simulink model "car_model_with_controller_2020a"  (R2020b)
settings: Solver=ode45  StartTime=0.0  StopTime=170  RelTol=1e-3
values from neighbouring files (symbols this model uses):
  d = 1.1    [constants.m]    (also in navigation.m = 0.64)
  Energy_budget = 1000*input("Define the energy budget(Kj): ")    [constants.m]
  J = 0.0025    [constants.m]
  Kb = 0.06    [constants.m]
  kd = 0    [constants.m]
  ki = 100    [constants.m]
  kp = 70    [constants.m]
  Kt = 11.43    [constants.m]
  l = 0.64    [constants.m]
  L = 0.125    [constants.m]    (also in navigation.m = 2.2)
  m = 810    [constants.m]
  N = 1000    [constants.m]
  P0 = 20    [constants.m]
  r = 0.256    [constants.m]    (also in navigation.m)
  R = 0.688    [constants.m]    (also in kin_controller.m = @(theta) [cos(theta),sin(theta),0;-sin(theta),cos(theta),0;0)
  T = trajectory.tSamples(2)    [constants.m]
  theta_init = atan2(ydot,xdot)    [constants.m]
  x_final = trajectory.q(1,end)    [constants.m]
  x_init = trajectory.q(1,1)    [constants.m]
  y_final = trajectory.q(2,end)    [constants.m]
  y_init = trajectory.q(2,1)    [constants.m]
libraries: simulink x2, pid_lib x2
settings Model: Creator=Tiago  LastModifiedBy=francisco
settings DebuggingCC: SFMachineParentedDataDiag=error  UnderSpecifiedDimensionMsg=warning

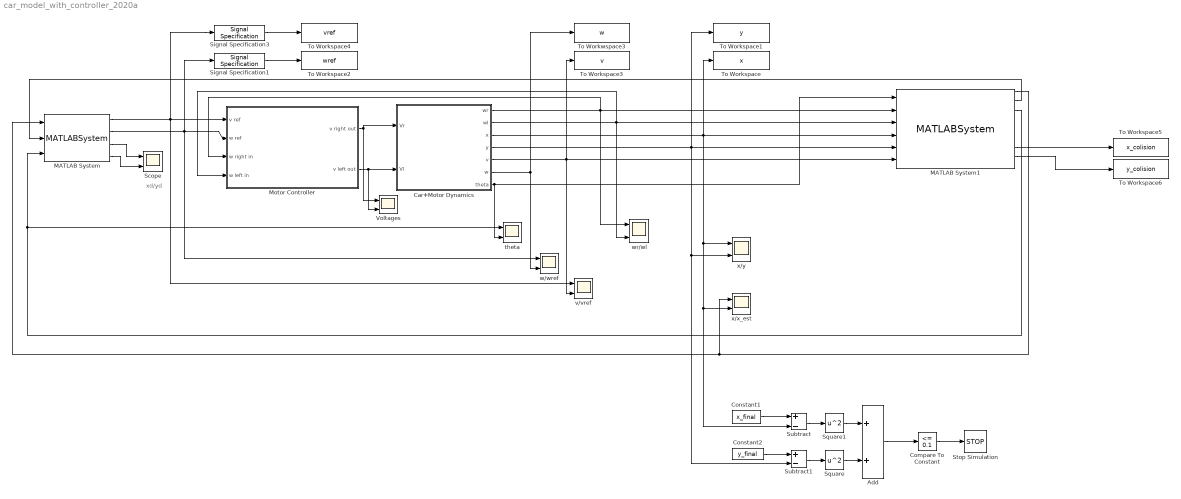
== system car_model_with_controller_2020a ==
  note: xd/yd
  Add : Sum
  Car+Motor Dynamics : Subsystem
  Compare To Constant : simulink/Logic and Bit Operations/Compare To Constant  relop=<=  const=0.1  OutDataTypeStr=boolean
  Constant1 : Constant  Value=x_final
  Constant2 : Constant  Value=y_final
  MATLAB System : MATLABSystem  System=kin_controller  traj=trajectory  OffsetTime=0.0  SampleTime=T  useKinematicModel=false  useFeedback=true  SimulateUsing=Code generation
      mask Type: kin_controller
      mask Display:
      | disp('kin_controller');
      | port_label('input',1,'x');
      | port_label('input',2,'y');
      | port_label('input',3,'theta');
      | port_label('output',1,'v');
      | port_label('output',2,'omega');
      | port_label('output',3,'xd');
      | port_label('output',4,'yd');
  MATLAB System1 : MATLABSystem  System=navigation  initial_x=x_init  initial_y=y_init  initial_theta=theta_init  q_gain=0.001  r_gain=5  OffsetTime=0.0  SampleTime=0.01  position_noise=2  orientation_noise=0.001  angular_speed_noise=0.001  oc_matx=oc_matx  d=0.64  L=2.2  Lr=0.566  Lf=0.566  k=0.1852  SimulateUsing=Code generation
      mask Type: navigation
      mask Display:
      | disp('navigation');
      | port_label('input',1,'theta_measured');
      | port_label('input',2,'omega_r');
      | port_label('input',3,'omega_l');
      | port_label('input',4,'x_real');
      | port_label('input',5,'y_real');
      | port_label('input',6,'V');
      | port_label('output',1,'x');
      | port_label('output',2,'y');
      | port_label('output',3,'theta');
      | port_label('output',4,'x_measured');
      | port_label('output',5,'y_measured');
      | port_label('output',6,'c_check');
      | port_label('output',7,'x_col');
      | port_label('output',8,'y_col');
      | port_label('output',9,'GPS');
  Motor Controller : Subsystem
  Scope : Scope  NumInputPorts=2
  Signal Specification1 : SignalSpecification  Dimensions=1
  Signal Specification3 : SignalSpecification  Dimensions=1
  Square : Math  Operator=square  SaturateOnIntegerOverflow=on
  Square1 : Math  Operator=square  SaturateOnIntegerOverflow=on
  Stop Simulation : Stop
  Subtract : Sum  Inputs=+-
  Subtract1 : Sum  Inputs=+-
  To Workspace : ToWorkspace  VariableName=x  SaveFormat=Timeseries  SampleTime=-1
  To Workspace1 : ToWorkspace  VariableName=y  SaveFormat=Timeseries  SampleTime=-1
  To Workspace2 : ToWorkspace  VariableName=wref  SaveFormat=Timeseries  SampleTime=-1
  To Workspace3 : ToWorkspace  VariableName=v  SaveFormat=Timeseries  SampleTime=-1
  To Workspace4 : ToWorkspace  VariableName=vref  SaveFormat=Timeseries  SampleTime=-1
  To Workspace5 : ToWorkspace  VariableName=x_colision  SampleTime=-1
      settings: Save2DSignal=2-D array (concatenate along first dimension)
  To Workspace6 : ToWorkspace  VariableName=y_colision  SampleTime=-1
      settings: Save2DSignal=2-D array (concatenate along first dimension)
  To Workwspace3 : ToWorkspace  VariableName=w  SaveFormat=Timeseries  SampleTime=-1
  Voltages : Scope  NumInputPorts=2
  theta : Scope  NumInputPorts=2
  v/vref : Scope  NumInputPorts=2
  w/wref : Scope  NumInputPorts=2
  wr/wl : Scope  NumInputPorts=2
  x/x_est : Scope  NumInputPorts=2
  x/y : Scope  NumInputPorts=2
  wires:
  Motor Controller/2(v left out) -> Car+Motor Dynamics/2(Vl), Voltages/2
  Motor Controller/1(v right out) -> Car+Motor Dynamics/1(Vr), Voltages/1
  MATLAB System1/3 -> MATLAB System/3, theta/1
  MATLAB System1/1 -> x/x_est/1, MATLAB System/1
  MATLAB System1/2 -> MATLAB System/2
  Car+Motor Dynamics/1(wr) -> wr/wl/1, MATLAB System1/2, Motor Controller/3(w right in)
  Car+Motor Dynamics/2(wl) -> wr/wl/2, MATLAB System1/3, Motor Controller/4(w left in)
  Car+Motor Dynamics/3(x) -> x/y/1, Subtract/2, x/x_est/2, MATLAB System1/4, To Workspace/1
  Car+Motor Dynamics/4(y) -> x/y/2, Subtract1/2, MATLAB System1/5, To Workspace1/1
  Car+Motor Dynamics/5(v) -> v/vref/2, MATLAB System1/6, To Workspace3/1
  Car+Motor Dynamics/6(w) -> w/wref/2, To Workwspace3/1
  Car+Motor Dynamics/7(theta) -> MATLAB System1/1, theta/2
  MATLAB System/1 -> v/vref/1, Motor Controller/1(v ref), Signal Specification3/1
  MATLAB System/2 -> w/wref/1, Signal Specification1/1, Motor Controller/2(w ref)
  MATLAB System/3 -> Scope/1
  MATLAB System/4 -> Scope/2
  Constant1/1 -> Subtract/1
  Constant2/1 -> Subtract1/1
  Subtract1/1 -> Square/1
  Subtract/1 -> Square1/1
  Compare To Constant/1 -> Stop Simulation/1
  Square1/1 -> Add/1
  Square/1 -> Add/2
  Add/1 -> Compare To Constant/1
  Signal Specification3/1 -> To Workspace4/1
  Signal Specification1/1 -> To Workspace2/1
  MATLAB System1/7 -> To Workspace5/1
  MATLAB System1/8 -> To Workspace6/1

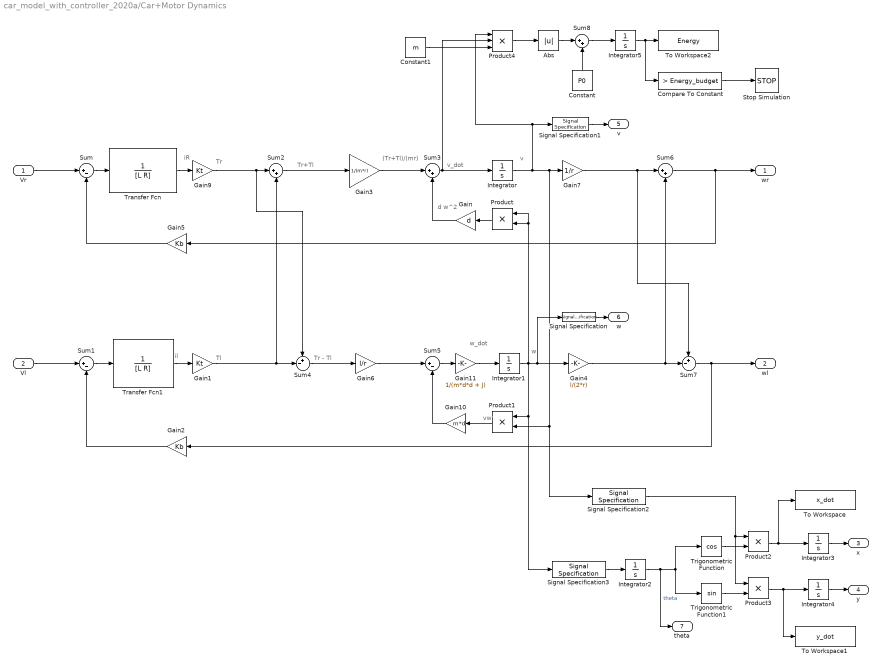
== system car_model_with_controller_2020a/Car+Motor Dynamics ==
  note: Tr+Tl
  note: w
  note: v_dot
  note: w_dot
  note: (Tr+Tl)/(mr)
  note: Tr
  note: iR
  note: v
  note: vw
  note: Tr - Tl
  note: il
  note: d w^2
  note: Tl
  Vr : Inport
  Vl : Inport  Port=2
  Abs : Abs
  Compare To Constant : simulink/Logic and Bit Operations/Compare To Constant  relop=>  const=Energy_budget  OutDataTypeStr=boolean
  Constant : Constant  Value=P0
  Constant1 : Constant  Value=m
  Gain : Gain  Gain=d
  Gain1 : Gain  Gain=Kt
  Gain10 : Gain  Gain=m*d
  Gain11 : Gain  Gain=1/(m*d*d + J)
  Gain2 : Gain  Gain=Kb
  Gain3 : Gain  Gain=1/(m*r)
  Gain4 : Gain  Gain=l/(2*r)
  Gain5 : Gain  Gain=Kb
  Gain6 : Gain  Gain=l/r
  Gain7 : Gain  Gain=1/r
  Gain9 : Gain  Gain=Kt
  Integrator : Integrator
  Integrator1 : Integrator
  Integrator2 : Integrator  InitialCondition=theta_init
  Integrator3 : Integrator  InitialCondition=x_init
  Integrator4 : Integrator  InitialCondition=y_init
  Integrator5 : Integrator
  Product{,1..3} (4 alike) : Product
  Product4 : Product  Inputs=3
  Signal Specification{,1..3} (4 alike) : SignalSpecification  Dimensions=1
  Stop Simulation : Stop
  Sum : Sum  Inputs=|+-
  Sum1 : Sum  Inputs=|+-
  Sum{2..3,6,8} (4 alike) : Sum  Inputs=|++
  Sum4 : Sum  Inputs=+-|
  Sum5 : Sum  Inputs=|+-
  Sum7 : Sum  Inputs=+-|
  To Workspace : ToWorkspace  VariableName=x_dot  SaveFormat=Timeseries  SampleTime=-1
  To Workspace1 : ToWorkspace  VariableName=y_dot  SaveFormat=Timeseries  SampleTime=-1
  To Workspace2 : ToWorkspace  VariableName=Energy  SaveFormat=Timeseries  SampleTime=-1
  Transfer Fcn : TransferFcn  Denominator=[L R]
  Transfer Fcn1 : TransferFcn  Denominator=[L R]
  Trigonometric Function : Trigonometry  Operator=cos
  Trigonometric Function1 : Trigonometry
  wr : Outport
  wl : Outport  Port=2
  x : Outport  Port=3
  y : Outport  Port=4
  v : Outport  Port=5
  w : Outport  Port=6
  theta : Outport  Port=7
  wires:
  Gain9/1 -> Sum4/1, Sum2/1
  Product/1 -> Gain/1
  Product3/1 -> To Workspace1/1, Integrator4/1
  Signal Specification2/1 -> Product3/1, Product2/1
  Sum3/1 -> Product4/2, Integrator/1
  Gain6/1 -> Sum5/1
  Gain2/1 -> Sum1/2
  Transfer Fcn/1 -> Gain9/1
  Transfer Fcn1/1 -> Gain1/1
  Gain5/1 -> Sum/2
  Signal Specification3/1 -> Integrator2/1
  Integrator1/1 -> Product/1, Product/2, Signal Specification/1, Gain4/1, Product1/1, Signal Specification3/1
  Gain10/1 -> Sum5/2
  Sum7/1 -> Gain2/1, wl/1
  Gain/1 -> Sum3/2
  Trigonometric Function/1 -> Product2/2
  Sum2/1 -> Gain3/1
  Vr/1 -> Sum/1
  Product2/1 -> To Workspace/1, Integrator3/1
  Gain3/1 -> Sum3/1
  Integrator2/1 -> theta/1, Trigonometric Function1/1, Trigonometric Function/1  "theta"
  Gain4/1 -> Sum7/2, Sum6/2
  Sum4/1 -> Gain6/1
  Integrator/1 -> Product4/1, Signal Specification1/1, Gain7/1, Signal Specification2/1, Product1/2
  Gain7/1 -> Sum6/1, Sum7/1
  Integrator3/1 -> x/1
  Signal Specification/1 -> w/1
  Vl/1 -> Sum1/1
  Signal Specification1/1 -> v/1
  Integrator4/1 -> y/1
  Sum1/1 -> Transfer Fcn1/1
  Gain1/1 -> Sum2/2, Sum4/2
  Sum5/1 -> Gain11/1
  Trigonometric Function1/1 -> Product3/2
  Sum6/1 -> wr/1, Gain5/1
  Gain11/1 -> Integrator1/1
  Product1/1 -> Gain10/1
  Sum/1 -> Transfer Fcn/1
  Sum8/1 -> Integrator5/1
  Abs/1 -> Sum8/1
  Product4/1 -> Abs/1
  Constant/1 -> Sum8/2
  Constant1/1 -> Product4/3
  Integrator5/1 -> Compare To Constant/1, To Workspace2/1
  Compare To Constant/1 -> Stop Simulation/1

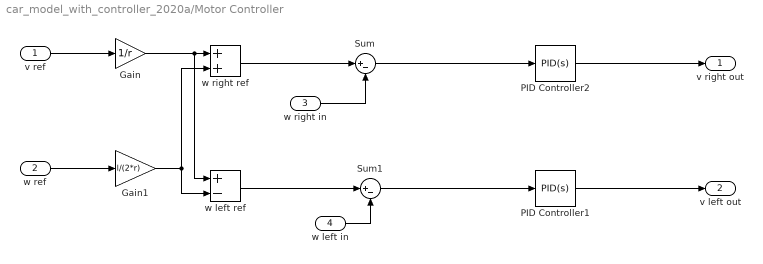
== system car_model_with_controller_2020a/Motor Controller ==
  v ref : Inport
  w ref : Inport  Port=2
  w right in : Inport  Port=3
  w left in : Inport  Port=4
  Gain : Gain  Gain=1/r
  Gain1 : Gain  Gain=l/(2*r)
  PID Controller1 : pid_lib/PID Controller  Controller=PID  Form=Parallel  TimeDomain=Continuous-time  UseExternalTs=off  SampleTime=-1  IntegratorMethod=Forward Euler  FilterMethod=Forward Euler  ControllerParametersSource=internal  P=kp  I=ki  D=kd  UseFilter=on  N=105296.504032148  TunerSelectOption=Transfer Function Based (PID Tuner App)  InitialConditionSource=internal  InitialConditionForIntegrator=0  InitialConditionForFilter=0  DifferentiatorICPrevScaledInput=0  ExternalReset=none  TrackingMode=off  Kt=1  LimitOutput=off  SatLimitsSource=internal  UpperSaturationLimit=inf  LowerSaturationLimit=-inf  LinearizeAsGain=on  AntiWindupMode=none  Kb=1  POutMin=[]  POutMax=[]  IOutMin=[]  IOutMax=[]  DOutMin=[]  DOutMax=[]  NOutMin=[]  NOutMax=[]  SumOutMin=[]  SumOutMax=[]  SaturationOutMin=[]  SaturationOutMax=[]  PParamMin=[]  PParamMax=[]  IParamMin=[]  IParamMax=[]  DParamMin=[]  DParamMax=[]  NParamMin=[]  NParamMax=[]  KbParamMin=[]  KbParamMax=[]  KtParamMin=[]  KtParamMax=[]  KbOutMin=[]  KbOutMax=[]  KtOutMin=[]  KtOutMax=[]  IntegratorOutMin=[]  IntegratorOutMax=[]  FilterOutMin=[]  FilterOutMax=[]  SumI1OutMin=[]  SumI1OutMax=[]  SumI2OutMin=[]  SumI2OutMax=[]  SumI3OutMin=[]  SumI3OutMax=[]  SumI4OutMin=[]  SumI4OutMax=[]  SumDOutMin=[]  SumDOutMax=[]  DifferentiatorOutMin=[]  DifferentiatorOutMax=[]  FilterDiffOutCoefMin=[]  FilterDiffOutCoefMax=[]  ReciprocalOutMin=[]  ReciprocalOutMax=[]  SumDenOutMin=[]  SumDenOutMax=[]  SumNumOutMin=[]  SumNumOutMax=[]  DivideOutMin=[]  DivideOutMax=[]  UdiffTsProdOutMin=[]  UdiffTsProdOutMax=[]  NTsProdOutMin=[]  NTsProdOutMax=[]  UintegralTsProdOutMin=[]  UintegralTsProdOutMax=[]  UngainTsProdOutMin=[]  UngainTsProdOutMax=[]  IntegratorContinuousStateAttributes=''  IntegratorStateMustResolveToSignalObject=off  IntegratorRTWStateStorageClass=Auto  FilterContinuousStateAttributes=''  FilterStateMustResolveToSignalObject=off  FilterRTWStateStorageClass=Auto  ParallelPVariant=InternalParameters  IdealPVariant=Disabled  IVariant=InternalParameters  DVariant=InternalParameters  IntegratorVariant=Continuous  SatVariant=Disabled  AWVariant=Passthrough  PCopyVariant=Disabled  TRVariant=Disabled  FdbkBlocksVariant=Forward  IdealPFdbkVariant=Disabled  SatFdbkVariant=Disabled  DerivativeFilterVariant=ContFilter  NVariant=InternalParameters  NCopyVariant=Disabled  FilterICVariant=InternalICsFilter  IntegratorICVariant=InternalICs  ExternalResetVariant=Disabled  TRSumVariant=Passthrough  SumFdbkVariant=Disabled  SumVariant=Sum_PID  TsampFilterVariant=InternalTs  TsampNgainVariant=Passthrough  TsampIntegralVariant=Passthrough  ExternalSaturationOutDataTypeStr=Inherit: Same as second input
  PID Controller2 : pid_lib/PID Controller  Controller=PID  Form=Parallel  TimeDomain=Continuous-time  UseExternalTs=off  SampleTime=-1  IntegratorMethod=Forward Euler  FilterMethod=Forward Euler  ControllerParametersSource=internal  P=ki  I=kp  D=kd  UseFilter=on  N=N  TunerSelectOption=Transfer Function Based (PID Tuner App)  InitialConditionSource=internal  InitialConditionForIntegrator=0  InitialConditionForFilter=0  DifferentiatorICPrevScaledInput=0  ExternalReset=none  TrackingMode=off  Kt=1  LimitOutput=off  SatLimitsSource=internal  UpperSaturationLimit=inf  LowerSaturationLimit=-inf  LinearizeAsGain=on  AntiWindupMode=none  Kb=1  POutMin=[]  POutMax=[]  IOutMin=[]  IOutMax=[]  DOutMin=[]  DOutMax=[]  NOutMin=[]  NOutMax=[]  SumOutMin=[]  SumOutMax=[]  SaturationOutMin=[]  SaturationOutMax=[]  PParamMin=[]  PParamMax=[]  IParamMin=[]  IParamMax=[]  DParamMin=[]  DParamMax=[]  NParamMin=[]  NParamMax=[]  KbParamMin=[]  KbParamMax=[]  KtParamMin=[]  KtParamMax=[]  KbOutMin=[]  KbOutMax=[]  KtOutMin=[]  KtOutMax=[]  IntegratorOutMin=[]  IntegratorOutMax=[]  FilterOutMin=[]  FilterOutMax=[]  SumI1OutMin=[]  SumI1OutMax=[]  SumI2OutMin=[]  SumI2OutMax=[]  SumI3OutMin=[]  SumI3OutMax=[]  SumI4OutMin=[]  SumI4OutMax=[]  SumDOutMin=[]  SumDOutMax=[]  DifferentiatorOutMin=[]  DifferentiatorOutMax=[]  FilterDiffOutCoefMin=[]  FilterDiffOutCoefMax=[]  ReciprocalOutMin=[]  ReciprocalOutMax=[]  SumDenOutMin=[]  SumDenOutMax=[]  SumNumOutMin=[]  SumNumOutMax=[]  DivideOutMin=[]  DivideOutMax=[]  UdiffTsProdOutMin=[]  UdiffTsProdOutMax=[]  NTsProdOutMin=[]  NTsProdOutMax=[]  UintegralTsProdOutMin=[]  UintegralTsProdOutMax=[]  UngainTsProdOutMin=[]  UngainTsProdOutMax=[]  IntegratorContinuousStateAttributes=''  IntegratorStateMustResolveToSignalObject=off  IntegratorRTWStateStorageClass=Auto  FilterContinuousStateAttributes=''  FilterStateMustResolveToSignalObject=off  FilterRTWStateStorageClass=Auto  ParallelPVariant=InternalParameters  IdealPVariant=Disabled  IVariant=InternalParameters  DVariant=InternalParameters  IntegratorVariant=Continuous  SatVariant=Disabled  AWVariant=Passthrough  PCopyVariant=Disabled  TRVariant=Disabled  FdbkBlocksVariant=Forward  IdealPFdbkVariant=Disabled  SatFdbkVariant=Disabled  DerivativeFilterVariant=ContFilter  NVariant=InternalParameters  NCopyVariant=Disabled  FilterICVariant=InternalICsFilter  IntegratorICVariant=InternalICs  ExternalResetVariant=Disabled  TRSumVariant=Passthrough  SumFdbkVariant=Disabled  SumVariant=Sum_PID  TsampFilterVariant=InternalTs  TsampNgainVariant=Passthrough  TsampIntegralVariant=Passthrough  ExternalSaturationOutDataTypeStr=Inherit: Same as second input
  Sum : Sum  Inputs=|+-
  Sum1 : Sum  Inputs=|+-
  w left ref : Sum  Inputs=+-
  w right ref : Sum
  v right out : Outport
  v left out : Outport  Port=2
  wires:
  Gain/1 -> w right ref/1, w left ref/1
  Gain1/1 -> w right ref/2, w left ref/2
  w right ref/1 -> Sum/1
  w left ref/1 -> Sum1/1
  w right in/1 -> Sum/2
  w left in/1 -> Sum1/2
  w ref/1 -> Gain1/1
  PID Controller2/1 -> v right out/1
  PID Controller1/1 -> v left out/1
  v ref/1 -> Gain/1
  Sum/1 -> PID Controller2/1
  Sum1/1 -> PID Controller1/1
